simulink model "ece456hw83cfg"  (R2017b)
settings: Solver=VariableStepAuto  StartTime=0.0  StopTime=6  RelTol=1e-3
values from neighbouring files (symbols this model uses):
  Kp = 1.65    [ece456hw7.m]    (also in ece456hw8.m = 14.8603130573)
  Td = .5*L    (= 0.56)    [ece456hw8.m]
  Ti = 2*L    (= 2.24)    [ece456hw8.m]
settings Model: Creator=b  LastModifiedBy=b

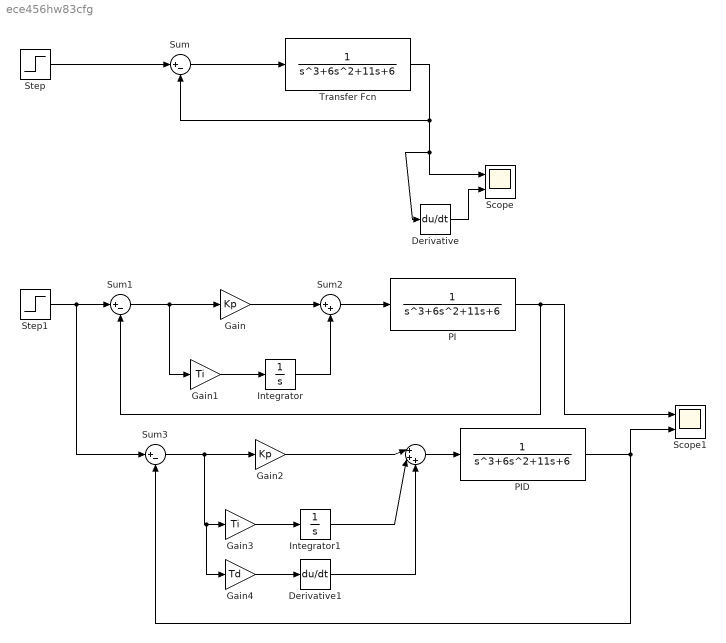
== system ece456hw83cfg ==
  " " : Sum  Inputs=|+++
  Derivative : Derivative
  Derivative1 : Derivative
  Gain : Gain  Gain=Kp
  Gain1 : Gain  Gain=Ti
  Gain2 : Gain  Gain=Kp
  Gain3 : Gain  Gain=Ti
  Gain4 : Gain  Gain=Td
  Integrator : Integrator
  Integrator1 : Integrator
  PI : TransferFcn  Denominator=[1 6 11 6]
  PID : TransferFcn  Denominator=[1 6 11 6]
  Scope : Scope  NumInputPorts=2
  Scope1 : Scope  NumInputPorts=2
  Step : Step  Before=1  SampleTime=0
  Step1 : Step  Before=1  SampleTime=0
  Sum : Sum  Inputs=|+-
  Sum1 : Sum  Inputs=|+-
  Sum2 : Sum  Inputs=|++
  Sum3 : Sum  Inputs=|+-
  Transfer Fcn : TransferFcn  Denominator=[1 6 11 6]
  wires:
  Sum/1 -> Transfer Fcn/1
  Transfer Fcn/1 -> Derivative/1, Scope/1, Sum/2
  Step/1 -> Sum/1
  Derivative/1 -> Scope/2
  Gain1/1 -> Integrator/1
  Sum1/1 -> Gain1/1, Gain/1
  Gain/1 -> Sum2/1
  Integrator/1 -> Sum2/2
  Step1/1 -> Sum3/1, Sum1/1
  Sum3/1 -> Gain4/1, Gain3/1, Gain2/1
  Gain3/1 -> Integrator1/1
  Integrator1/1 -> " "/2
  Gain2/1 -> " "/1
  Gain4/1 -> Derivative1/1
  Derivative1/1 -> " "/3
  Sum2/1 -> PI/1
  PI/1 -> Sum1/2, Scope1/1
  " "/1 -> PID/1
  PID/1 -> Sum3/2, Scope1/2
